simulink model "Perfect_blend_delayed_Quadcopter_Simulation"  (R2017a)
settings: Solver=ode45  StartTime=0.0  StopTime=35  FixedStep=0.05  MaxStep=0.06  RelTol=1e-3  EnableMultiTasking=on
model workspace (MAT data in the model file):
  Sig = Simulink.Signal
  Sig.DataType = 'auto'
  Sig.Dimensions = -1
  Sig.DimensionsMode = 'auto'
  Sig.Complexity = 'auto'
  Sig.SampleTime = -1
  Sig.SamplingMode = 'auto'
undefined symbols (not defined in the file or in its folder): altitude_error, blend_trigger, current_blend, error1, error2, error3, error4, IC, quadModel
libraries: simulink x4
(part 1 of 2)
Description:
  | This is a configurable quadcopter simulation.
  | This Simulink model demonstates position control.
  | 
  | Additional quadcopter modeling and simulation materials available at:
  | github.com/dch33/Quad-Sim
  | 
  | Copyright (C) 2014 D. Hartman, K. Landis, S. Moreno, J. Kim, M. Mehrer
  | 
  | License:
  |     This program is free software: you can redistribute it and/or modify
  |     it under the terms of the GNU LESSER GENERAL PUBLIC LICENSE as published by
  |     the Free Software Foundation, either version 3 of the License, or
  |     (at your option) any later version.
  | 
  |     This program is distributed in the hope that it will be useful,
  |     but WITHOUT ANY WARRANTY; without even the implied warranty of
  |     MERCHANTABILITY or FITNESS FOR A PARTICULAR PURPOSE.  See the
  |     GNU General Public License for more details.
  | 
  |     You should have received a copy of the GNU LESSER GENERAL PUBLIC LICENSE
  |     along with this program.  If not, see <http://www.gnu.org/licenses/>.
settings Model: ModifiedComment=davidhartman -- Fri Jun 06 22:59:54 2014 -- Version 1.5  Creator=David Hartman  LastModifiedBy=Yves
settings Model: ModifiedHistory=|
  | davidhartman -- Fri Jun 06 22:59:54 2014 -- Version 1.5
  | 
  | 
  | davidhartman -- Fri Jun 06 22:59:54 2014 -- Version 1.5
settings DataIOCC: ExternalInput=[Phi_sim_blend, Theta_sim_blend, Psi_sim_blend, error1, error2, error3, error4,]  FinalStateName=sim_result_final  InitialState=sim_state  SaveFormat=Array  SignalLogging=off  StateSaveName=sim_out_states  ReturnWorkspaceOutputsName=sim_all_outputs
settings OptimizationCC: DefaultParameterBehavior=Inlined  LifeSpan=inf
settings DebuggingCC: SolverPrmCheckMsg=warning  UniqueDataStoreMsg=warning  StateNameClashWarn=warning  StrictBusMsg=ErrorOnBusTreatedAsVector  SFUnexpectedBacktrackingDiag=warning  SFNoUnconditionalDefaultTransitionDiag=warning  SFExecutionAtInitializationDiag=none
settings HardwareCC: ProdBitPerPointer=32  ProdBitPerSizeT=32  ProdBitPerPtrDiffT=32  ProdLargestAtomicFloat=None  ProdIntDivRoundTo=Undefined  ProdEndianess=Unspecified  ProdWordSize=32  ProdHWDeviceType=32-bit Generic
settings ModelReferenceCC: PropagateSignalLabelsOutOfModel=off
settings GRTTargetCC: TargetLangStandard=C89/C90 (ANSI)  GeneratePreprocessorConditionals=Disable all
settings ConfigComp: CovMetricSettings=dw  CovHtmlReporting=on  CovSaveCumulativeToWorkspaceVar=on  CovSaveSingleToWorkspaceVar=on  CovExternalEMLEnable=off

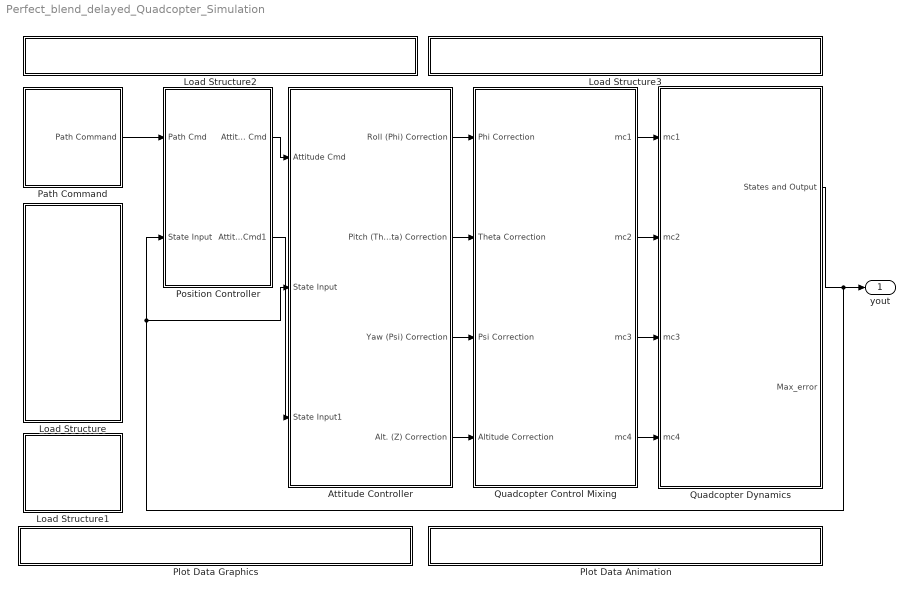
== system Perfect_blend_delayed_Quadcopter_Simulation ==
  Attitude Controller : Subsystem
  Load Structure : Subsystem
      settings: OpenFcn=|
      | uiopen('load')
      | if ((exist('IC')==1) && (exist('quadModel')==1) && (exist('path')==1))
      | set_param(bdroot, 'SimulationCommand', 'update')
      | end
      mask Display: fprintf('LOAD:\nTimeseries\nPath\nCommands,\nQuadcopter\nModel, Or\nInitial\nConditions');
  Load Structure1 : Subsystem
      settings: OpenFcn=|
      | if (exist('IC')==1 && exist('quadModel')==1 && exist('yout') && exist('tout'))
      | saveSimResults()
      | else
      | msgbox('No Data To Save!')
      | end
      mask Display: fprintf('SAVE:\nSimulation\nResults');
  Load Structure2 : Subsystem
      settings: OpenFcn=|
      | if exist('GUI_Modeling') == 2,
      | run('GUI_Modeling')
      | 
      | else
      | 
      | msgbox('The desired GUI must be first added to MATLABs path.')
      | 
      | end
      mask Display: fprintf('OPEN GUI: Build New \n Model');
  Load Structure3 : Subsystem
      settings: OpenFcn=|
      | if exist('GUI_IC') == 2,
      | run('GUI_IC')
      | 
      | else
      | 
      | msgbox('The desired GUI must be first added to MATLABs path.')
      | 
      | end
      mask Display: fprintf('OPEN GUI: Create Initial \n Conditions');
  Path Command : Subsystem  mask{Interpolate=on, OutputAfterFinalValue=Holding final value}
      mask prompts: Interpolate "Interpolate X, Y, Z, and Psi command data?"; OutputAfterFinalValue "Form output after final data value by:"
      mask help:
      | Selecting the Interpolate data checkbox causes position commands to be
      | linearly interpolated. For additional options related to the Timeseries
      | "path" commands, look under the block and click on the Timeseries From
      | Workspace blocks.
      mask TypeOptions Interpolate: X Timeseries From Wkspace/Interpolate | Y Timeseries From Wkspace/Interpolate | Z Timeseries From Wkspace/Interpolate | Psi Timeseries From Wkspace/Interpolate
      mask TypeOptions OutputAfterFinalValue: X Timeseries From Wkspace/OutputAfterFinalValue | Y Timeseries From Wkspace/OutputAfterFinalValue | Z Timeseries From Wkspace/OutputAfterFinalValue | Psi Timeseries From Wkspace/OutputAfterFinalValue
  Plot Data Animation : Subsystem
      settings: OpenFcn=|
      | if exist('QuadAnim4') == 2,
      |     if exist('yout')
      | 	run('QuadAnim4');
      |     else
      |     msgbox('Simulation must be run before data can be plotted.');
      |     end
      | else                                                                          msgbox('The desired GUI must be first added to MATLABs path.')
      | end
      mask Display: fprintf('OPEN GUI: Flight Animation')
  Plot Data Graphics : Subsystem
      settings: OpenFcn=|
      | if exist('yout')
      | yout = evalin('base', 'yout');
      | tout = evalin('base', 'tout');
      | quadPlots(yout, tout)
      | else
      | msgbox('Simulation must be run before data can be plotted.')
      | end
      mask Display: fprintf('OPEN PLOT: State Data')
  Position Controller : Subsystem
  Quadcopter Control Mixing : Subsystem
      mask Display:
      | modelLoaded = evalin('base','exist(''quadModel'',''var'')');
      | if (modelLoaded==1)
      |     if (evalin('base','quadModel.plusConfig'))
      |     fprintf([' \n' ' \n'  'Configuration "+"']);
      |     else if (~evalin('base','quadModel.plusConfig'))
      |         fprintf([' \n' ' \n' 'Configuration "X"']);
      |         end
      |     end
      | else
      |     fprintf([' \n' ' \n'  'Model Not Loaded']);
      | end
  Quadcopter Dynamics : Subsystem
  yout : Outport
  wires:
  Quadcopter Control Mixing/1(mc1) -> Quadcopter Dynamics/1(mc1)
  Quadcopter Control Mixing/2(mc2) -> Quadcopter Dynamics/2(mc2)
  Quadcopter Control Mixing/3(mc3) -> Quadcopter Dynamics/3(mc3)
  Quadcopter Control Mixing/4(mc4) -> Quadcopter Dynamics/4(mc4)
  Quadcopter Dynamics/1(States and Output) -> yout/1, Position Controller/2(State Input), Attitude Controller/2(State Input)
  Attitude Controller/1(Roll (Phi) Correction) -> Quadcopter Control Mixing/1(Phi Correction)
  Attitude Controller/2(Pitch (Theta) Correction) -> Quadcopter Control Mixing/2(Theta Correction)
  Attitude Controller/3(Yaw (Psi) Correction) -> Quadcopter Control Mixing/3(Psi Correction)
  Attitude Controller/4(Alt. (Z) Correction) -> Quadcopter Control Mixing/4(Altitude Correction)
  Path Command/1("Path Command ") -> Position Controller/1(Path Cmd)
  Position Controller/1(Attitude Cmd) -> Attitude Controller/1(Attitude Cmd)
  Position Controller/2(Attitude Cmd1) -> Attitude Controller/3(State Input1)

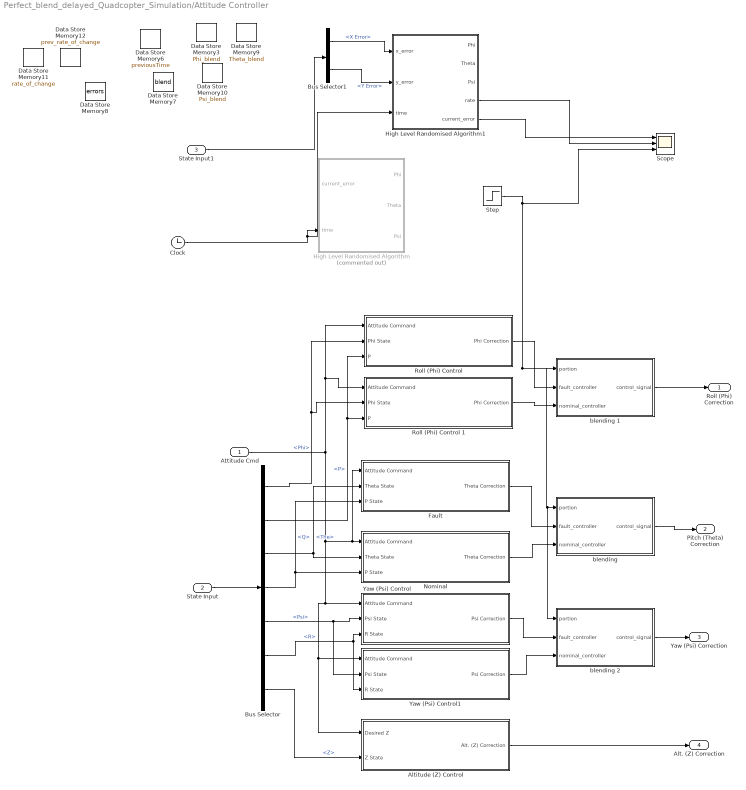
== system Perfect_blend_delayed_Quadcopter_Simulation/Attitude Controller ==
  Attitude Cmd : Inport
  State Input : Inport  Port=2
  State Input1 : Inport  Port=3
  Altitude (Z) Control : Subsystem  mask{Kpz=2, Kiz=1.1, Kdz=3.3, LimitOutput=on, USat=1, LSat=-1, GOffset=(sqrt((quadModel.mass*quadModel.g)/(4*quadModel.ct))-quadModel.b)/quadModel.cr}
      mask prompts: Kpz "Kp"; Kiz "Ki"; Kdz "Kd"; LimitOutput "Integral Saturation?"; USat "Upper saturation limit:"; LSat "Lower saturation limit:"; GOffset "Gravity Feedforward"
      mask help:
      | Adjust PID controller gains through this mask interface, or "look under mask" for more detailed adjustments.
      |
      | Note: Gravity Offset will not appear on block face as a value until simulation is run if it is the result of a formula involving the quadcopter model parameters.
      mask TypeOptions Kpz: Kpz/Gain
      mask TypeOptions Kiz: Kiz/Gain
      mask TypeOptions Kdz: Kdz/Gain
      mask TypeOptions LimitOutput:
      | Integrator
      | Limited/LimitOutput
      mask TypeOptions USat:
      | Integrator
      | Limited/UpperSaturationLimit
      mask TypeOptions LSat:
      | Integrator
      | Limited/LowerSaturationLimit
      mask TypeOptions GOffset: Gravity Offset (Level Flight)/Value
      mask Display:
      | fprintf(['Gravity Offset = ' num2str(GOffset) '\n' ...
      |     'Kp = ' num2str(Kpz) '\n' ...
      |     'Ki = ' num2str(Kiz) '\n' ...
      |     'Kd = ' num2str(Kdz) '\n' ...
      |     'Integral Saturation: ' LimitOutput]);
      | if strcmp(LimitOutput,'on')
      |     fprintf([' \n' ' \n' ' \n' ' \n' ' \n' '\n' ...
      |         'Limits: ' num2str(USat) ' to ' num2str(LSat)]);
      | end
  Bus Selector : BusSelector  OutputSignals=Phi,P,The,Q,Psi,R,Z
  Bus Selector1 : BusSelector  OutputSignals=X Error,Y Error
  Clock : Clock
  Data Store Memory10 : DataStoreMemory  DataStoreName=Psi_blend  ReadBeforeWriteMsg=warning  WriteAfterWriteMsg=warning  WriteAfterReadMsg=warning  ShowAdditionalParam=off  OutDataTypeStr=double
  Data Store Memory11 : DataStoreMemory  DataStoreName=rate_of_change  ReadBeforeWriteMsg=warning  WriteAfterWriteMsg=warning  WriteAfterReadMsg=warning  ShowAdditionalParam=off  OutDataTypeStr=double
  Data Store Memory12 : DataStoreMemory  DataStoreName=prev_rate_of_change  ReadBeforeWriteMsg=warning  WriteAfterWriteMsg=warning  WriteAfterReadMsg=warning  ShowAdditionalParam=off  OutDataTypeStr=double
  Data Store Memory3 : DataStoreMemory  DataStoreName=Phi_blend  ReadBeforeWriteMsg=warning  WriteAfterWriteMsg=warning  WriteAfterReadMsg=warning  ShowAdditionalParam=off  OutDataTypeStr=double
  Data Store Memory6 : DataStoreMemory  DataStoreName=previousTime  ReadBeforeWriteMsg=warning  WriteAfterWriteMsg=warning  WriteAfterReadMsg=warning  ShowAdditionalParam=off  OutDataTypeStr=double  Dimensions=[5 1]
  Data Store Memory7 : DataStoreMemory  DataStoreName=blend  ReadBeforeWriteMsg=warning  WriteAfterWriteMsg=warning  WriteAfterReadMsg=warning  ShowAdditionalParam=off  OutDataTypeStr=double
  Data Store Memory8 : DataStoreMemory  DataStoreName=errors  ReadBeforeWriteMsg=warning  WriteAfterWriteMsg=warning  WriteAfterReadMsg=warning  ShowAdditionalParam=off  OutDataTypeStr=double  Dimensions=[5 1]
  Data Store Memory9 : DataStoreMemory  DataStoreName=Theta_blend  ReadBeforeWriteMsg=warning  WriteAfterWriteMsg=warning  WriteAfterReadMsg=warning  ShowAdditionalParam=off  OutDataTypeStr=double
  Fault : Subsystem  mask{Kpt=10, Kit=5, Kdt=3, LimitOutput=on, USat=1, LSat=-1}
      mask prompts: Kpt "Kp"; Kit "Ki"; Kdt "Kd"; LimitOutput "Integral Saturation?"; USat "Upper saturation limit:"; LSat "Lower saturation limit:"
      mask help: Adjust PID controller gains through this mask interface, or "look under mask" for more detailed adjustments.
      mask TypeOptions Kpt: Kpt/Gain
      mask TypeOptions Kit: Kit/Gain
      mask TypeOptions Kdt: Kdt/Gain
      mask TypeOptions LimitOutput:
      | Integrator
      | Limited/LimitOutput
      mask TypeOptions USat:
      | Integrator
      | Limited/UpperSaturationLimit
      mask TypeOptions LSat:
      | Integrator
      | Limited/LowerSaturationLimit
      mask Display:
      | fprintf(['Kp = ' num2str(Kpt) '\n' ...
      |     'Ki = ' num2str(Kit) '\n' ...
      |     'Kd = ' num2str(Kdt) '\n' ...
      |     'Integral Saturation: ' LimitOutput]);
      | if strcmp(LimitOutput,'on')
      |     fprintf([' \n' ' \n' ' \n' ' \n' '\n' ...
      |         'Limits: ' num2str(USat) ' to ' num2str(LSat)]);
      | end
  High Level Randomised Algorithm : MATLAB Function  Commented=on  TreatAsAtomicUnit=on
  High Level Randomised Algorithm1 : MATLAB Function  TreatAsAtomicUnit=on
  Nominal : Subsystem  mask{Kpt=2, Kit=1.1, Kdt=1.2, LimitOutput=on, USat=1, LSat=-1}
      mask prompts: Kpt "Kp"; Kit "Ki"; Kdt "Kd"; LimitOutput "Integral Saturation?"; USat "Upper saturation limit:"; LSat "Lower saturation limit:"
      mask help: Adjust PID controller gains through this mask interface, or "look under mask" for more detailed adjustments.
      mask TypeOptions Kpt: Kpt/Gain
      mask TypeOptions Kit: Kit/Gain
      mask TypeOptions Kdt: Kdt/Gain
      mask TypeOptions LimitOutput:
      | Integrator
      | Limited/LimitOutput
      mask TypeOptions USat:
      | Integrator
      | Limited/UpperSaturationLimit
      mask TypeOptions LSat:
      | Integrator
      | Limited/LowerSaturationLimit
      mask Display:
      | fprintf(['Kp = ' num2str(Kpt) '\n' ...
      |     'Ki = ' num2str(Kit) '\n' ...
      |     'Kd = ' num2str(Kdt) '\n' ...
      |     'Integral Saturation: ' LimitOutput]);
      | if strcmp(LimitOutput,'on')
      |     fprintf([' \n' ' \n' ' \n' ' \n' '\n' ...
      |         'Limits: ' num2str(USat) ' to ' num2str(LSat)]);
      | end
  "Roll (Phi) Control " : Subsystem  mask{Kpp=10, Kip=5, Kdp=3, LimitOutput=on, USat=1, LSat=-1}
      mask prompts: Kpp "Kp"; Kip "Ki"; Kdp "Kd"; LimitOutput "Integral Saturation:"; USat "Upper saturation limit:"; LSat "Lower saturation limit:"
      mask help:
      | Adjust PID controller gains through this mask interface, or "look under mask"
      | for more detailed adjustments.
      mask TypeOptions Kpp: Kpp/Gain
      mask TypeOptions Kip: Kip/Gain
      mask TypeOptions Kdp: Kdp/Gain
      mask TypeOptions LimitOutput:
      | Integrator
      | Limited/LimitOutput
      mask TypeOptions USat:
      | Integrator
      | Limited/UpperSaturationLimit
      mask TypeOptions LSat:
      | Integrator
      | Limited/LowerSaturationLimit
      mask Display:
      | fprintf(['Kp = ' num2str(Kpp) '\n' ...
      |     'Ki = ' num2str(Kip) '\n' ...
      |     'Kd = ' num2str(Kdp) '\n'...
      |     'Integral Saturation: ' LimitOutput]);
      | if strcmp(LimitOutput,'on')
      |     fprintf([' \n' ' \n' ' \n' ' \n' '\n' ...
      |         'Limits: ' num2str(USat) ' to ' num2str(LSat)]);
      | end
  Roll (Phi) Control 1 : Subsystem  mask{Kpp=2.0, Kip=1.1, Kdp=1.2, LimitOutput=on, USat=1, LSat=-1}
      mask prompts: Kpp "Kp"; Kip "Ki"; Kdp "Kd"; LimitOutput "Integral Saturation:"; USat "Upper saturation limit:"; LSat "Lower saturation limit:"
      mask help:
      | Adjust PID controller gains through this mask interface, or "look under mask"
      | for more detailed adjustments.
      mask TypeOptions Kpp: Kpp/Gain
      mask TypeOptions Kip: Kip/Gain
      mask TypeOptions Kdp: Kdp/Gain
      mask TypeOptions LimitOutput:
      | Integrator
      | Limited/LimitOutput
      mask TypeOptions USat:
      | Integrator
      | Limited/UpperSaturationLimit
      mask TypeOptions LSat:
      | Integrator
      | Limited/LowerSaturationLimit
      mask Display:
      | fprintf(['Kp = ' num2str(Kpp) '\n' ...
      |     'Ki = ' num2str(Kip) '\n' ...
      |     'Kd = ' num2str(Kdp) '\n'...
      |     'Integral Saturation: ' LimitOutput]);
      | if strcmp(LimitOutput,'on')
      |     fprintf([' \n' ' \n' ' \n' ' \n' '\n' ...
      |         'Limits: ' num2str(USat) ' to ' num2str(LSat)]);
      | end
  Scope : Scope  NumInputPorts=3
  Step : Step  Time=blend_trigger  After=current_blend  SampleTime=0
  Yaw (Psi) Control : Subsystem  mask{Kps=12, Kis=2, Kds=5, LimitOutput=on, USat=1, LSat=-1}
      mask prompts: Kps "Kp"; Kis "Ki"; Kds "Kd"; LimitOutput "Integral Saturation?"; USat "Upper saturation limit:"; LSat "Lower saturation limit:"
      mask help: Adjust PID controller gains through this mask interface, or "look under mask" for more detailed adjustments.
      mask TypeOptions Kps: Kps/Gain
      mask TypeOptions Kis: Kit/Gain
      mask TypeOptions Kds: Kds/Gain
      mask TypeOptions LimitOutput:
      | Integrator
      | Limited/LimitOutput
      mask TypeOptions USat:
      | Integrator
      | Limited/UpperSaturationLimit
      mask TypeOptions LSat:
      | Integrator
      | Limited/LowerSaturationLimit
      mask Display:
      | fprintf(['Kp = ' num2str(Kps) '\n' ...
      |     'Ki = ' num2str(Kis) '\n' ...
      |     'Kd = ' num2str(Kds) '\n' ...
      |     'Integral Saturation: ' LimitOutput]);
      | if strcmp(LimitOutput,'on')
      |     fprintf([' \n' ' \n' ' \n' ' \n' '\n' ...
      |         'Limits: ' num2str(USat) ' to ' num2str(LSat)]);
      | end
  Yaw (Psi) Control1 : Subsystem  mask{Kps=4, Kis=0.5, Kds=3.5, LimitOutput=on, USat=1, LSat=-1}
      mask prompts: Kps "Kp"; Kis "Ki"; Kds "Kd"; LimitOutput "Integral Saturation?"; USat "Upper saturation limit:"; LSat "Lower saturation limit:"
      mask help: Adjust PID controller gains through this mask interface, or "look under mask" for more detailed adjustments.
      mask TypeOptions Kps: Kps/Gain
      mask TypeOptions Kis: Kit/Gain
      mask TypeOptions Kds: Kds/Gain
      mask TypeOptions LimitOutput:
      | Integrator
      | Limited/LimitOutput
      mask TypeOptions USat:
      | Integrator
      | Limited/UpperSaturationLimit
      mask TypeOptions LSat:
      | Integrator
      | Limited/LowerSaturationLimit
      mask Display:
      | fprintf(['Kp = ' num2str(Kps) '\n' ...
      |     'Ki = ' num2str(Kis) '\n' ...
      |     'Kd = ' num2str(Kds) '\n' ...
      |     'Integral Saturation: ' LimitOutput]);
      | if strcmp(LimitOutput,'on')
      |     fprintf([' \n' ' \n' ' \n' ' \n' '\n' ...
      |         'Limits: ' num2str(USat) ' to ' num2str(LSat)]);
      | end
  "blending " : MATLAB Function  TreatAsAtomicUnit=on
  blending 1 : MATLAB Function  TreatAsAtomicUnit=on
  blending 2 : MATLAB Function  TreatAsAtomicUnit=on
  Roll (Phi) Correction : Outport
  Pitch (Theta) Correction : Outport  Port=2
  Yaw (Psi) Correction : Outport  Port=3
  Alt. (Z) Correction : Outport  Port=4
  wires:
  Bus Selector/1 -> Roll (Phi) Control 1/2(Phi State), "Roll (Phi) Control "/2(Phi State)  "<Phi>"
  State Input/1 -> Bus Selector/1
  Bus Selector/5 -> Yaw (Psi) Control1/2(Psi State), Yaw (Psi) Control/2(Psi State)  "<Psi>"
  Altitude (Z) Control/1(Alt. (Z) Correction) -> Alt. (Z) Correction/1
  Bus Selector/7 -> Altitude (Z) Control/2(Z State)  "<Z>"
  Attitude Cmd/1 -> Yaw (Psi) Control1/1(Attitude Command), Altitude (Z) Control/1(Desired Z), Yaw (Psi) Control/1(Attitude Command), Fault/1(Attitude Command), Nominal/1(Attitude Command), Roll (Phi) Control 1/1("Attitude Command "), "Roll (Phi) Control "/1("Attitude Command ")
  Bus Selector/3 -> Nominal/2(Theta State), Fault/2(Theta State)  "<The>"
  Bus Selector/2 -> Roll (Phi) Control 1/3(P), "Roll (Phi) Control "/3(P)  "<P>"
  Bus Selector/4 -> Fault/3(P State), Nominal/3(P State)  "<Q>"
  Bus Selector/6 -> Yaw (Psi) Control1/3(R State), Yaw (Psi) Control/3(R State)  "<R>"
  Nominal/1(Theta Correction) -> "blending "/3(nominal_controller)
  Fault/1(Theta Correction) -> "blending "/2(fault_controller)
  "blending "/1(control_signal) -> Pitch (Theta) Correction/1
  Roll (Phi) Control 1/1(Phi Correction) -> blending 1/3(nominal_controller)
  "Roll (Phi) Control "/1(Phi Correction) -> blending 1/2(fault_controller)
  blending 1/1(control_signal) -> Roll (Phi) Correction/1
  Yaw (Psi) Control/1(Psi Correction) -> blending 2/2(fault_controller)
  Yaw (Psi) Control1/1(Psi Correction) -> blending 2/3(nominal_controller)
  blending 2/1(control_signal) -> Yaw (Psi) Correction/1
  Clock/1 -> High Level Randomised Algorithm1/3(time), High Level Randomised Algorithm/2(time)
  Step/1 -> Scope/3, blending 2/1(portion), "blending "/1(portion), blending 1/1(portion)
  Bus Selector1/2 -> High Level Randomised Algorithm1/2(y_error)  "<Y Error>"
  Bus Selector1/1 -> High Level Randomised Algorithm1/1(x_error)  "<X Error>"
  State Input1/1 -> Bus Selector1/1
  High Level Randomised Algorithm1/4(rate) -> Scope/2
  High Level Randomised Algorithm1/5(current_error) -> Scope/1

== system Perfect_blend_delayed_Quadcopter_Simulation/Load Structure ==

== system Perfect_blend_delayed_Quadcopter_Simulation/Load Structure1 ==

== system Perfect_blend_delayed_Quadcopter_Simulation/Load Structure2 ==

== system Perfect_blend_delayed_Quadcopter_Simulation/Load Structure3 ==

== system Perfect_blend_delayed_Quadcopter_Simulation/Path Command ==
  Bus Creator : BusCreator  Inputs=4
  Bus Selector : BusSelector  OutputSignals=X_cmd,Y_cmd  OutputAsBus=on
  Psi Timeseries From Wkspace : FromWorkspace  VariableName=path.psi  SampleTime=0  OutputAfterFinalValue=Holding final value
  X Timeseries From Wkspace : FromWorkspace  VariableName=path.x  SampleTime=0  OutputAfterFinalValue=Holding final value
  Y Timeseries From Wkspace : FromWorkspace  VariableName=path.y  SampleTime=0  OutputAfterFinalValue=Holding final value
  Z Timeseries From Wkspace : FromWorkspace  VariableName=path.z  SampleTime=0  OutputAfterFinalValue=Holding final value
  "Path Command " : Outport
  tag scope: C=global
  wires:
  X Timeseries From Wkspace/1 -> Bus Creator/1  "X_cmd"
  Y Timeseries From Wkspace/1 -> Bus Creator/2  "Y_cmd"
  Z Timeseries From Wkspace/1 -> Bus Creator/3  "Alt_Cmd"
  Psi Timeseries From Wkspace/1 -> Bus Creator/4  "Psi_cmd"
  Bus Creator/1 -> Bus Selector/1, "Path Command "/1  "Path_Cmd"
  Bus Selector/1 -> [C]  "XY_Cmd"

== system Perfect_blend_delayed_Quadcopter_Simulation/Plot Data Animation ==

== system Perfect_blend_delayed_Quadcopter_Simulation/Plot Data Graphics ==

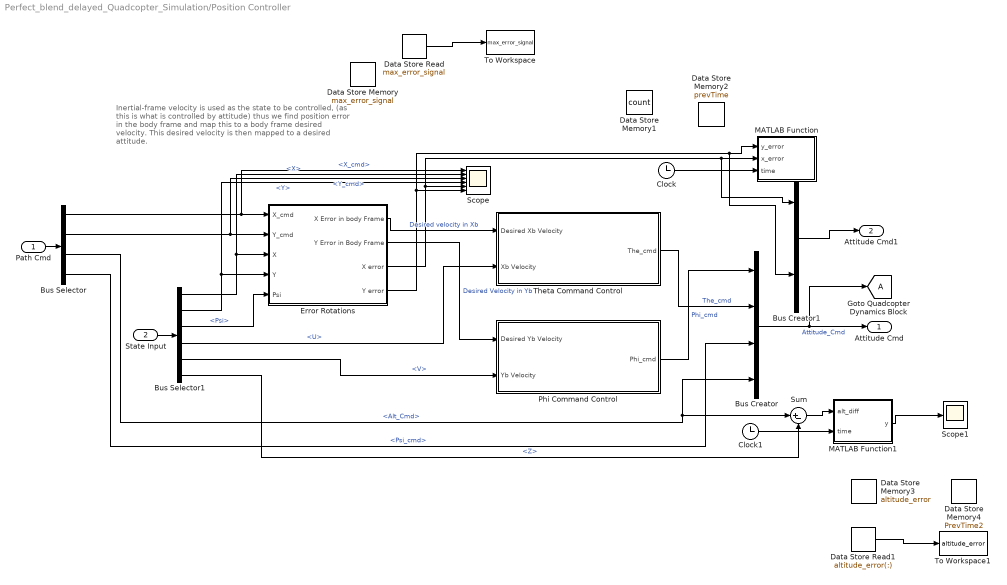
== system Perfect_blend_delayed_Quadcopter_Simulation/Position Controller ==
  note: Inertial-frame velocity is used as the state to be controlled,
      | (as this is what is controlled by attitude)
      | thus we find position error in the body frame
      | and map this to a body frame desired velocity. This desired
      | velocity is then mapped to a desired attitude.
  Path Cmd : Inport
  State Input : Inport  Port=2
  Bus Creator : BusCreator  Inputs=4
  Bus Creator1 : BusCreator  Inputs=2
  Bus Selector : BusSelector  OutputSignals=X_cmd,Y_cmd,Alt_Cmd,Psi_cmd
  Bus Selector1 : BusSelector  OutputSignals=X,Y,Psi,U,V,Z
  Clock : Clock
  Clock1 : Clock
  Data Store Memory : DataStoreMemory  DataStoreName=max_error_signal  ReadBeforeWriteMsg=warning  WriteAfterWriteMsg=warning  WriteAfterReadMsg=warning  ShowAdditionalParam=off  OutDataTypeStr=double
  Data Store Memory1 : DataStoreMemory  DataStoreName=count  ReadBeforeWriteMsg=warning  WriteAfterWriteMsg=warning  WriteAfterReadMsg=warning  ShowAdditionalParam=off  OutDataTypeStr=double
  Data Store Memory2 : DataStoreMemory  DataStoreName=prevTime  ReadBeforeWriteMsg=warning  WriteAfterWriteMsg=warning  WriteAfterReadMsg=warning  ShowAdditionalParam=off  OutDataTypeStr=double
  Data Store Memory3 : DataStoreMemory  DataStoreName=altitude_error  ReadBeforeWriteMsg=warning  WriteAfterWriteMsg=warning  WriteAfterReadMsg=warning  ShowAdditionalParam=off  OutDataTypeStr=double
  Data Store Memory4 : DataStoreMemory  DataStoreName=PrevTime2  ReadBeforeWriteMsg=warning  WriteAfterWriteMsg=warning  WriteAfterReadMsg=warning  ShowAdditionalParam=off  OutDataTypeStr=double
  Data Store Read : DataStoreRead  DataStoreName=max_error_signal  DataStoreElements=max_error_signal
  Data Store Read1 : DataStoreRead  DataStoreName=altitude_error  DataStoreElements=altitude_error(:)
  Error Rotations : Subsystem
  MATLAB Function : MATLAB Function  TreatAsAtomicUnit=on
  MATLAB Function1 : MATLAB Function  TreatAsAtomicUnit=on
  Phi Command Control : Subsystem  mask{Kp=0.32, Kd=0.1, ASat=12*pi/180}
      mask prompts: Kp "Proportional Gain"; Kd "Derivative Gain"; ASat "Attitude Limit (+/- radians):"
      mask TypeOptions Kp: Kpp/Gain
      mask TypeOptions Kd: Kdp/Gain
      mask TypeOptions ASat: Attitude Limits_Phi/UpperLimit
      mask Display:
      | fprintf(['Kp = ' num2str(Kp) '\n' ...
      |     'Kd = ' num2str(Kd) '\n' ...
      |     'Attitude Limit (+/-): ' num2str(ASat*180/pi) '°']);
  Scope : Scope  NumInputPorts=6
  Scope1 : Scope
  Sum : Sum  Inputs=|+-
  Theta Command Control : Subsystem  mask{Kp=0.32, Kd=0.10, ASat=12*pi/180}
      mask prompts: Kp "Proportional Gain:"; Kd "Derivative Gain"; ASat "Attitude Limit (+/- radians):"
      mask TypeOptions Kp: Kpt/Gain
      mask TypeOptions Kd: Kdt/Gain
      mask TypeOptions ASat: Attitude Limits_Theta/UpperLimit
      mask Display:
      | fprintf(['Kp = ' num2str(Kp) '\n' ...
      |     'Kd = ' num2str(Kd) '\n' ...
      |     'Attitude Limit (+/-): ' num2str(ASat*180/pi) '°']);
  To Workspace : ToWorkspace  VariableName=max_error_signal  SampleTime=-1
      settings: MaxDataPoints=1
  To Workspace1 : ToWorkspace  VariableName=altitude_error  SampleTime=-1
      settings: MaxDataPoints=1
  Attitude Cmd : Outport
  Attitude Cmd1 : Outport  Port=2
  tag scope: A=global
  wires:
  Bus Selector1/5 -> Phi Command Control/2(Yb Velocity)  "<V>"
  State Input/1 -> Bus Selector1/1
  Bus Selector/4 -> Bus Creator/3  "<Psi_cmd>"
  Path Cmd/1 -> Bus Selector/1
  Bus Selector/3 -> Sum/1, Bus Creator/4  "<Alt_Cmd>"
  Bus Creator/1 -> Attitude Cmd/1, [A]  "Attitude_Cmd"
  Bus Selector/1 -> Scope/1, Error Rotations/1(X_cmd)  "<X_cmd>"
  Bus Selector/2 -> Error Rotations/2(Y_cmd), Scope/3  "<Y_cmd>"
  Bus Selector1/1 -> Error Rotations/3(X), Scope/2  "<X>"
  Bus Selector1/2 -> Error Rotations/4(Y), Scope/4  "<Y>"
  Bus Selector1/3 -> Error Rotations/5(Psi)  "<Psi>"
  Error Rotations/1(X Error in body Frame) -> Theta Command Control/1(Desired Xb Velocity)  "Desired velocity in Xb"
  Bus Selector1/4 -> Theta Command Control/2(Xb Velocity)  "<U>"
  Theta Command Control/1(The_cmd) -> Bus Creator/2  "The_cmd"
  Error Rotations/2(Y Error in Body Frame) -> Phi Command Control/1(Desired Yb Velocity)  "Desired Velocity in Yb"
  Phi Command Control/1(Phi_cmd) -> Bus Creator/1  "Phi_cmd"
  Data Store Read/1 -> To Workspace/1
  Error Rotations/3(X error) -> Bus Creator1/1, MATLAB Function/2(x_error), Scope/5
  Error Rotations/4("Y error ") -> Bus Creator1/2, MATLAB Function/1(y_error), Scope/6
  Clock/1 -> MATLAB Function/3(time)
  MATLAB Function1/1(y) -> Scope1/1
  Data Store Read1/1 -> To Workspace1/1
  Sum/1 -> MATLAB Function1/1(alt_diff)
  Bus Selector1/6 -> Sum/2  "<Z>"
  Clock1/1 -> MATLAB Function1/2(time)
  Bus Creator1/1 -> Attitude Cmd1/1

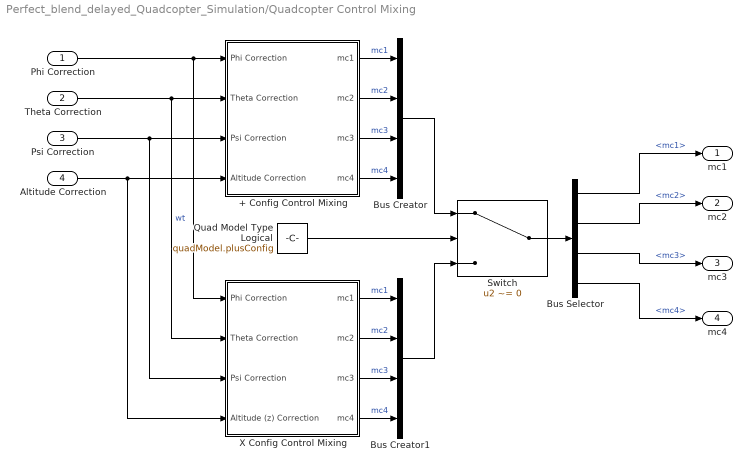
== system Perfect_blend_delayed_Quadcopter_Simulation/Quadcopter Control Mixing ==
  Phi Correction : Inport
  Theta Correction : Inport  Port=2
  Psi Correction : Inport  Port=3
  Altitude Correction : Inport  Port=4
  + Config Control Mixing : Subsystem
  Bus Creator : BusCreator  Inputs=4
  Bus Creator1 : BusCreator  Inputs=4
  Bus Selector : BusSelector  OutputSignals=mc1,mc2,mc3,mc4
  Quad Model Type Logical : Constant  Value=quadModel.plusConfig
  Switch : Switch  Criteria=u2 ~= 0
  X Config Control Mixing : Subsystem
  mc1 : Outport
  mc2 : Outport  Port=2
  mc3 : Outport  Port=3
  mc4 : Outport  Port=4
  wires:
  Phi Correction/1 -> X Config Control Mixing/1(Phi Correction), + Config Control Mixing/1(Phi Correction)
  Theta Correction/1 -> X Config Control Mixing/2(Theta Correction), + Config Control Mixing/2(Theta Correction)  "wt"
  Psi Correction/1 -> X Config Control Mixing/3(Psi Correction), + Config Control Mixing/3(Psi Correction)
  Altitude Correction/1 -> X Config Control Mixing/4(Altitude (z) Correction), + Config Control Mixing/4(Altitude Correction)
  + Config Control Mixing/1(mc1) -> Bus Creator/1  "mc1"
  + Config Control Mixing/2(mc2) -> Bus Creator/2  "mc2"
  + Config Control Mixing/3(mc3) -> Bus Creator/3  "mc3"
  + Config Control Mixing/4(mc4) -> Bus Creator/4  "mc4"
  Bus Creator/1 -> Switch/1
  X Config Control Mixing/1(mc1) -> Bus Creator1/1  "mc1"
  X Config Control Mixing/2(mc2) -> Bus Creator1/2  "mc2"
  X Config Control Mixing/3(mc3) -> Bus Creator1/3  "mc3"
  X Config Control Mixing/4(mc4) -> Bus Creator1/4  "mc4"
  Bus Creator1/1 -> Switch/3
  Bus Selector/1 -> mc1/1  "<mc1>"
  Bus Selector/2 -> mc2/1  "<mc2>"
  Bus Selector/3 -> mc3/1  "<mc3>"
  Bus Selector/4 -> mc4/1  "<mc4>"
  Quad Model Type Logical/1 -> Switch/2
  Switch/1 -> Bus Selector/1

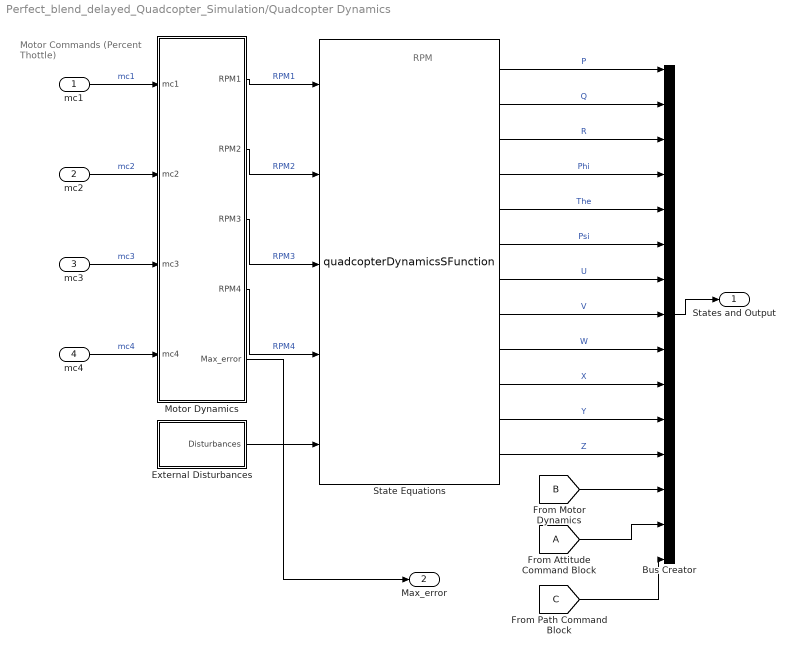
== system Perfect_blend_delayed_Quadcopter_Simulation/Quadcopter Dynamics ==
  note: RPM
  note: Motor Commands
      | (Percent Thottle)
  mc1 : Inport
  mc2 : Inport  Port=2
  mc3 : Inport  Port=3
  mc4 : Inport  Port=4
  Bus Creator : BusCreator  Inputs='P','Q','R','Phi','The','Psi','U','V','W','X','Y','Z','mc and RPM','Attitude_Cmd','XY_Cmd'
  External Disturbances : Subsystem
  Motor Dynamics : Subsystem
  State Equations : M-S-Function  FunctionName=quadcopterDynamicsSFunction  Parameters=quadModel, IC
      mask Display:
      | port_label('input', 1, 'RPM1')
      | port_label('input', 2, 'RPM2')
      | port_label('input', 3, 'RPM3')
      | port_label('input', 4, 'RPM4')
      | port_label('input', 5, 'Disturbances')
      | port_label('output', 1, 'P')
      | port_label('output', 2, 'Q')
      | port_label('output', 3, 'R')
      | port_label('output', 4, 'Phi')
      | port_label('output', 5, 'The')
      | port_label('output', 6, 'Psi')
      | port_label('output', 7, 'U')
      | port_label('output', 8, 'V')
      | port_label('output', 9, 'W')
      | port_label('output', 10, 'X')
      | port_label('output', 11, 'Y')
      | port_label('output', 12, 'Z')
  States and Output : Outport
  "Max_error " : Outport  Port=2
  wires:
  State Equations/1 -> Bus Creator/1  "P"
  State Equations/2 -> Bus Creator/2  "Q"
  State Equations/3 -> Bus Creator/3  "R"
  State Equations/4 -> Bus Creator/4  "Phi"
  State Equations/5 -> Bus Creator/5  "The"
  State Equations/6 -> Bus Creator/6  "Psi"
  State Equations/7 -> Bus Creator/7  "U"
  State Equations/8 -> Bus Creator/8  "V"
  State Equations/9 -> Bus Creator/9  "W"
  State Equations/10 -> Bus Creator/10  "X"
  State Equations/11 -> Bus Creator/11  "Y"
  State Equations/12 -> Bus Creator/12  "Z"
  Bus Creator/1 -> States and Output/1
  Motor Dynamics/1(RPM1) -> State Equations/1  "RPM1"
  Motor Dynamics/2(RPM2) -> State Equations/2  "RPM2"
  Motor Dynamics/3(RPM3) -> State Equations/3  "RPM3"
  Motor Dynamics/4(RPM4) -> State Equations/4  "RPM4"
  mc1/1 -> Motor Dynamics/1(mc1)  "mc1"
  mc4/1 -> Motor Dynamics/4(mc4)  "mc4"
  mc3/1 -> Motor Dynamics/3(mc3)  "mc3"
  mc2/1 -> Motor Dynamics/2(mc2)  "mc2"
  External Disturbances/1("Disturbances ") -> State Equations/5
  [A] -> Bus Creator/14
  [B] -> Bus Creator/13
  [C] -> Bus Creator/15
  Motor Dynamics/5("Max_error ") -> "Max_error "/1

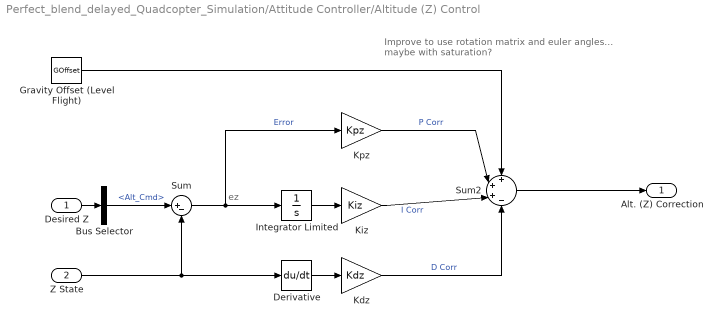
== system Perfect_blend_delayed_Quadcopter_Simulation/Attitude Controller/Altitude (Z) Control ==
  note: Improve to use rotation matrix and euler angles...
      | maybe with saturation?
  note: ez
  Desired Z : Inport
  Z State : Inport  Port=2
  Bus Selector : BusSelector  OutputSignals=Alt_Cmd
  Derivative : Derivative
  Gravity Offset (Level Flight) : Constant  Value=GOffset
  Integrator Limited : Integrator  LimitOutput=on  UpperSaturationLimit=USat  LowerSaturationLimit=LSat
  Kdz : Gain  Gain=Kdz
  Kiz : Gain  Gain=Kiz
  Kpz : Gain  Gain=Kpz
  Sum : Sum  Inputs=|+-
  Sum2 : Sum  Inputs=+++-
  Alt. (Z) Correction : Outport
  wires:
  Gravity Offset (Level Flight)/1 -> Sum2/1
  Desired Z/1 -> Bus Selector/1
  Z State/1 -> Derivative/1, Sum/2
  Sum2/1 -> Alt. (Z) Correction/1
  Kpz/1 -> Sum2/2  "P Corr"
  Sum/1 -> Integrator Limited/1, Kpz/1  "Error"
  Kiz/1 -> Sum2/3  "I Corr"
  Kdz/1 -> Sum2/4  "D Corr"
  Integrator Limited/1 -> Kiz/1
  Bus Selector/1 -> Sum/1  "<Alt_Cmd>"
  Derivative/1 -> Kdz/1

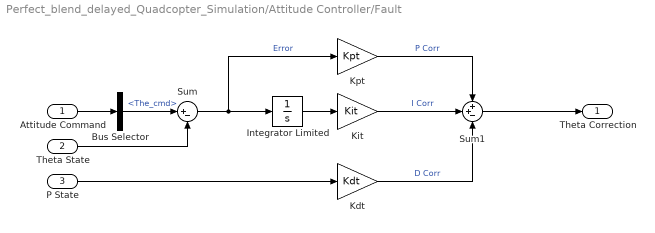
== system Perfect_blend_delayed_Quadcopter_Simulation/Attitude Controller/Fault ==
  Attitude Command : Inport
  Theta State : Inport  Port=2
  P State : Inport  Port=3
  Bus Selector : BusSelector  OutputSignals=The_cmd
  Integrator Limited : Integrator  LimitOutput=on  UpperSaturationLimit=USat  LowerSaturationLimit=LSat
  Kdt : Gain  Gain=Kdt
  Kit : Gain  Gain=Kit
  Kpt : Gain  Gain=Kpt
  Sum : Sum  Inputs=|+-
  Sum1 : Sum  Inputs=++-
  Theta Correction : Outport
  wires:
  Sum/1 -> Integrator Limited/1, Kpt/1  "Error"
  Attitude Command/1 -> Bus Selector/1
  Theta State/1 -> Sum/2
  Sum1/1 -> Theta Correction/1
  Kpt/1 -> Sum1/1  "P Corr"
  Kdt/1 -> Sum1/3  "D Corr"
  Kit/1 -> Sum1/2  "I Corr"
  Integrator Limited/1 -> Kit/1
  Bus Selector/1 -> Sum/1  "<The_cmd>"
  P State/1 -> Kdt/1

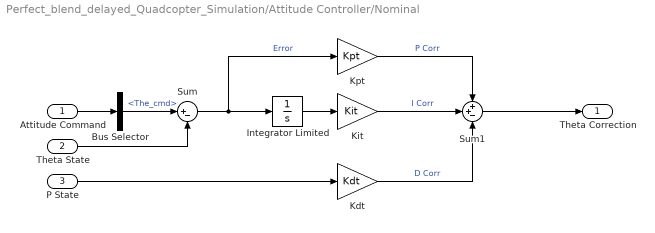
== system Perfect_blend_delayed_Quadcopter_Simulation/Attitude Controller/Nominal ==
  Attitude Command : Inport
  Theta State : Inport  Port=2
  P State : Inport  Port=3
  Bus Selector : BusSelector  OutputSignals=The_cmd
  Integrator Limited : Integrator  LimitOutput=on  UpperSaturationLimit=USat  LowerSaturationLimit=LSat
  Kdt : Gain  Gain=Kdt
  Kit : Gain  Gain=Kit
  Kpt : Gain  Gain=Kpt
  Sum : Sum  Inputs=|+-
  Sum1 : Sum  Inputs=++-
  Theta Correction : Outport
  wires:
  Sum/1 -> Integrator Limited/1, Kpt/1  "Error"
  Attitude Command/1 -> Bus Selector/1
  Theta State/1 -> Sum/2
  Sum1/1 -> Theta Correction/1
  Kpt/1 -> Sum1/1  "P Corr"
  Kdt/1 -> Sum1/3  "D Corr"
  Kit/1 -> Sum1/2  "I Corr"
  Integrator Limited/1 -> Kit/1
  Bus Selector/1 -> Sum/1  "<The_cmd>"
  P State/1 -> Kdt/1

== system Perfect_blend_delayed_Quadcopter_Simulation/Attitude Controller/Roll (Phi) Control  ==
  "Attitude Command " : Inport
  Phi State : Inport  Port=2
  P : Inport  Port=3
  Bus Selector : BusSelector  OutputSignals=Phi_cmd
  Integrator Limited : Integrator  LimitOutput=on  UpperSaturationLimit=USat  LowerSaturationLimit=LSat
  Kdp : Gain  Gain=Kdp
  Kip : Gain  Gain=Kip
  Kpp : Gain  Gain=Kpp
  Sum : Sum  Inputs=|+-
  Sum1 : Sum  Inputs=++-
  Phi Correction : Outport
  wires:
  Sum/1 -> Integrator Limited/1, Kpp/1  "Error"
  Phi State/1 -> Sum/2
  Sum1/1 -> Phi Correction/1
  Kpp/1 -> Sum1/1  "P Corr"
  Kdp/1 -> Sum1/3  "D Corr"
  Kip/1 -> Sum1/2  "I Corr"
  Integrator Limited/1 -> Kip/1
  "Attitude Command "/1 -> Bus Selector/1
  Bus Selector/1 -> Sum/1  "<Phi_cmd>"
  P/1 -> Kdp/1

== system Perfect_blend_delayed_Quadcopter_Simulation/Attitude Controller/Roll (Phi) Control 1 ==
  "Attitude Command " : Inport
  Phi State : Inport  Port=2
  P : Inport  Port=3
  Bus Selector : BusSelector  OutputSignals=Phi_cmd
  Integrator Limited : Integrator  LimitOutput=on  UpperSaturationLimit=USat  LowerSaturationLimit=LSat
  Kdp : Gain  Gain=Kdp
  Kip : Gain  Gain=Kip
  Kpp : Gain  Gain=Kpp
  Sum : Sum  Inputs=|+-
  Sum1 : Sum  Inputs=++-
  Phi Correction : Outport
  wires:
  P/1 -> Kdp/1
  Bus Selector/1 -> Sum/1  "<Phi_cmd>"
  "Attitude Command "/1 -> Bus Selector/1
  Integrator Limited/1 -> Kip/1
  Kip/1 -> Sum1/2  "I Corr"
  Kdp/1 -> Sum1/3  "D Corr"
  Kpp/1 -> Sum1/1  "P Corr"
  Sum1/1 -> Phi Correction/1
  Phi State/1 -> Sum/2
  Sum/1 -> Kpp/1, Integrator Limited/1  "Error"

== system Perfect_blend_delayed_Quadcopter_Simulation/Attitude Controller/Yaw (Psi) Control ==
  Attitude Command : Inport
  Psi State : Inport  Port=2
  R State : Inport  Port=3
  Bus Selector : BusSelector  OutputSignals=Psi_cmd
  Integrator Limited : Integrator  LimitOutput=on  UpperSaturationLimit=USat  LowerSaturationLimit=LSat
  Kds : Gain  Gain=Kds
  Kit : Gain  Gain=Kis
  Kps : Gain  Gain=Kps
  Sum : Sum  Inputs=|+-
  Sum1 : Sum  Inputs=++-
  Psi Correction : Outport
  wires:
  Sum/1 -> Integrator Limited/1, Kps/1  "Error"
  Attitude Command/1 -> Bus Selector/1
  Sum1/1 -> Psi Correction/1
  Psi State/1 -> Sum/2
  Kps/1 -> Sum1/1  "P Corr"
  Kds/1 -> Sum1/3  "D Corr"
  Kit/1 -> Sum1/2  "I Corr"
  Integrator Limited/1 -> Kit/1
  Bus Selector/1 -> Sum/1  "<Psi_cmd>"
  R State/1 -> Kds/1

== system Perfect_blend_delayed_Quadcopter_Simulation/Attitude Controller/Yaw (Psi) Control1 ==
  Attitude Command : Inport
  Psi State : Inport  Port=2
  R State : Inport  Port=3
  Bus Selector : BusSelector  OutputSignals=Psi_cmd
  Integrator Limited : Integrator  LimitOutput=on  UpperSaturationLimit=USat  LowerSaturationLimit=LSat
  Kds : Gain  Gain=Kds
  Kit : Gain  Gain=Kis
  Kps : Gain  Gain=Kps
  Sum : Sum  Inputs=|+-
  Sum1 : Sum  Inputs=++-
  Psi Correction : Outport
  wires:
  Sum/1 -> Integrator Limited/1, Kps/1  "Error"
  Attitude Command/1 -> Bus Selector/1
  Sum1/1 -> Psi Correction/1
  Psi State/1 -> Sum/2
  Kps/1 -> Sum1/1  "P Corr"
  Kds/1 -> Sum1/3  "D Corr"
  Kit/1 -> Sum1/2  "I Corr"
  Integrator Limited/1 -> Kit/1
  Bus Selector/1 -> Sum/1  "<Psi_cmd>"
  R State/1 -> Kds/1

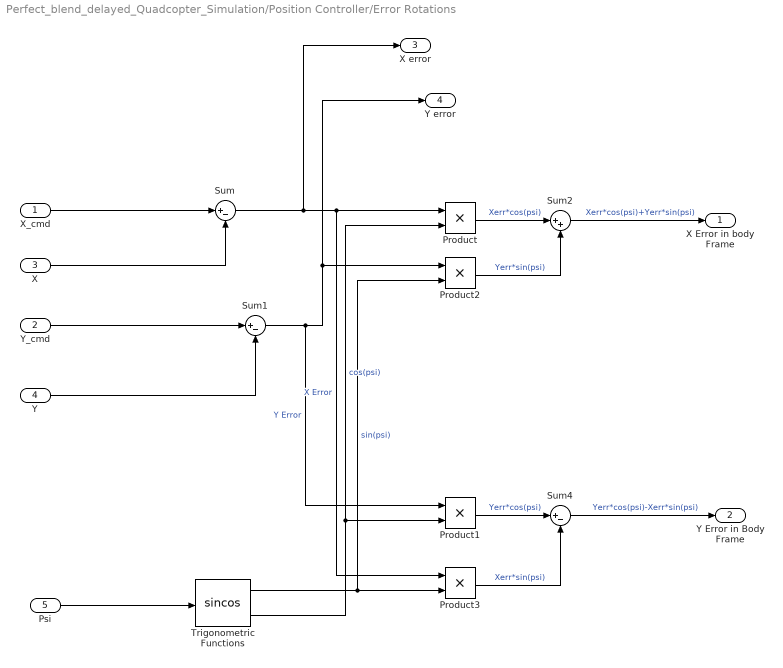
== system Perfect_blend_delayed_Quadcopter_Simulation/Position Controller/Error Rotations ==
  X_cmd : Inport
  Y_cmd : Inport  Port=2
  X : Inport  Port=3
  Y : Inport  Port=4
  Psi : Inport  Port=5
  Product{,1..3} (4 alike) : Product
  Sum : Sum  Inputs=|+-
  Sum1 : Sum  Inputs=|+-
  Sum2 : Sum  Inputs=|++
  Sum4 : Sum  Inputs=|+-
  Trigonometric Functions : Trigonometry  Operator=sincos
  X Error in body Frame : Outport
  Y Error in Body Frame : Outport  Port=2
  X error : Outport  Port=3
  "Y error " : Outport  Port=4
  wires:
  Sum4/1 -> Y Error in Body Frame/1  "Yerr*cos(psi)-Xerr*sin(psi)"
  Product3/1 -> Sum4/2  "Xerr*sin(psi)"
  Sum1/1 -> "Y error "/1, Product2/1, Product1/1  "Y Error"
  Trigonometric Functions/1 -> Product2/2, Product3/2  "sin(psi)"
  Sum2/1 -> X Error in body Frame/1  "Xerr*cos(psi)+Yerr*sin(psi)"
  Y_cmd/1 -> Sum1/1
  X_cmd/1 -> Sum/1
  X/1 -> Sum/2
  Y/1 -> Sum1/2
  Sum/1 -> X error/1, Product3/1, Product/1  "X Error"
  Trigonometric Functions/2 -> Product/2, Product1/2  "cos(psi)"
  Product/1 -> Sum2/1  "Xerr*cos(psi)"
  Product2/1 -> Sum2/2  "Yerr*sin(psi)"
  Product1/1 -> Sum4/1  "Yerr*cos(psi)"
  Psi/1 -> Trigonometric Functions/1

== system Perfect_blend_delayed_Quadcopter_Simulation/Position Controller/Phi Command Control ==
  note: -1 Gain is required because a "negative"
      | angle of Phi induces a positive velocity
      | in the body frame y direction!
  Desired Yb Velocity : Inport
  Yb Velocity : Inport  Port=2
  Attitude Limits_Phi : Saturate  UpperLimit=ASat  LowerLimit=-ASat
  Gain : Gain  Gain=-1
  Kdp : Gain  Gain=Kd
  Kpp : Gain  Gain=Kp
  Sum3 : Sum  Inputs=|+-
  Sum6 : Sum  Inputs=|+-
  V Derivative : Derivative
  Phi_cmd : Outport
  wires:
  V Derivative/1 -> Kdp/1
  Attitude Limits_Phi/1 -> Phi_cmd/1  "Phi_cmd"
  Sum6/1 -> Gain/1
  Kpp/1 -> Sum6/1
  Sum3/1 -> Kpp/1  "Velocity Error"
  Yb Velocity/1 -> V Derivative/1, Sum3/2
  Desired Yb Velocity/1 -> Sum3/1
  Gain/1 -> Attitude Limits_Phi/1
  Kdp/1 -> Sum6/2

== system Perfect_blend_delayed_Quadcopter_Simulation/Position Controller/Theta Command Control ==
  Desired Xb Velocity : Inport
  Xb Velocity : Inport  Port=2
  Attitude Limits_Theta : Saturate  UpperLimit=ASat  LowerLimit=-ASat
  Kdt : Gain  Gain=Kd
  Kpt : Gain  Gain=Kp
  Sum3 : Sum  Inputs=|+-
  Sum6 : Sum  Inputs=|+-
  U Derivative : Derivative
  The_cmd : Outport
  wires:
  Kdt/1 -> Sum6/2
  U Derivative/1 -> Kdt/1
  Attitude Limits_Theta/1 -> The_cmd/1  "The_cmd"
  Sum6/1 -> Attitude Limits_Theta/1
  Kpt/1 -> Sum6/1
  Sum3/1 -> Kpt/1  "Velocity Error"
  Xb Velocity/1 -> U Derivative/1, Sum3/2
  Desired Xb Velocity/1 -> Sum3/1

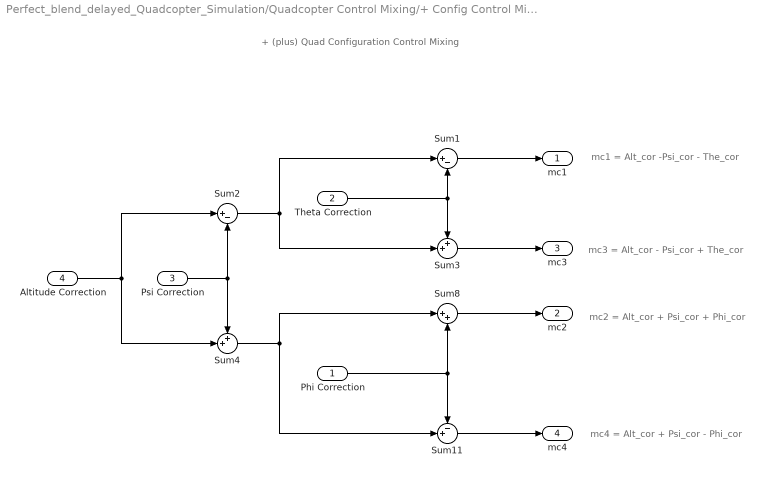
== system Perfect_blend_delayed_Quadcopter_Simulation/Quadcopter Control Mixing/+ Config Control Mixing ==
  note: mc2 = Alt_cor + Psi_cor + Phi_cor
  note: + (plus) Quad Configuration Control Mixing
  note: mc4 = Alt_cor + Psi_cor - Phi_cor
  note: mc3 = Alt_cor - Psi_cor + The_cor
  note: mc1 = Alt_cor -Psi_cor - The_cor
  Phi Correction : Inport
  Theta Correction : Inport  Port=2
  Psi Correction : Inport  Port=3
  Altitude Correction : Inport  Port=4
  Sum1 : Sum  Inputs=|+-
  Sum11 : Sum  Inputs=-+|
  Sum2 : Sum  Inputs=|+-
  Sum3 : Sum  Inputs=++|
  Sum4 : Sum  Inputs=++|
  Sum8 : Sum  Inputs=|++
  mc1 : Outport
  mc2 : Outport  Port=2
  mc3 : Outport  Port=3
  mc4 : Outport  Port=4
  wires:
  Altitude Correction/1 -> Sum2/1, Sum4/2
  Sum2/1 -> Sum3/2, Sum1/1
  Psi Correction/1 -> Sum4/1, Sum2/2
  Sum4/1 -> Sum11/2, Sum8/1
  Phi Correction/1 -> Sum8/2, Sum11/1
  Sum1/1 -> mc1/1
  Sum3/1 -> mc3/1
  Sum8/1 -> mc2/1
  Sum11/1 -> mc4/1
  Theta Correction/1 -> Sum1/2, Sum3/1

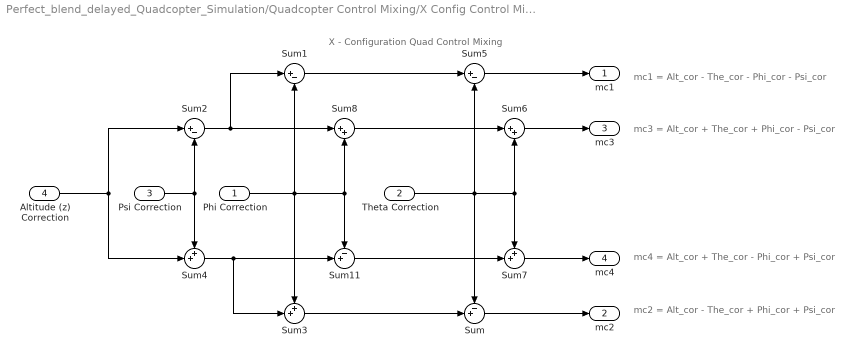
== system Perfect_blend_delayed_Quadcopter_Simulation/Quadcopter Control Mixing/X Config Control Mixing ==
  note: mc1 = Alt_cor - The_cor - Phi_cor - Psi_cor
  note: X - Configuration Quad Control Mixing
  note: mc3 = Alt_cor + The_cor + Phi_cor - Psi_cor
  note: mc2 = Alt_cor - The_cor + Phi_cor + Psi_cor
  note: mc4 = Alt_cor + The_cor - Phi_cor + Psi_cor
  Phi Correction : Inport
  Theta Correction : Inport  Port=2
  Psi Correction : Inport  Port=3
  Altitude (z) Correction : Inport  Port=4
  Sum : Sum  Inputs=-+|
  Sum1 : Sum  Inputs=|+-
  Sum11 : Sum  Inputs=-+|
  Sum2 : Sum  Inputs=|+-
  Sum3 : Sum  Inputs=++|
  Sum4 : Sum  Inputs=++|
  Sum5 : Sum  Inputs=|+-
  Sum6 : Sum  Inputs=|++
  Sum7 : Sum  Inputs=++|
  Sum8 : Sum  Inputs=|++
  mc1 : Outport
  mc2 : Outport  Port=2
  mc3 : Outport  Port=3
  mc4 : Outport  Port=4
  wires:
  Sum2/1 -> Sum8/1, Sum1/1
  Psi Correction/1 -> Sum4/1, Sum2/2
  Phi Correction/1 -> Sum3/1, Sum1/2, Sum8/2, Sum11/1
  Sum4/1 -> Sum3/2, Sum11/2
  Sum3/1 -> Sum/2
  Theta Correction/1 -> Sum7/1, Sum6/2, Sum5/2, Sum/1
  Sum1/1 -> Sum5/1
  Sum8/1 -> Sum6/1
  Sum11/1 -> Sum7/2
  Sum5/1 -> mc1/1
  Sum6/1 -> mc3/1
  Sum7/1 -> mc4/1
  Altitude (z) Correction/1 -> Sum2/1, Sum4/2
  Sum/1 -> mc2/1

== system Perfect_blend_delayed_Quadcopter_Simulation/Quadcopter Dynamics/External Disturbances ==
  note: Note: Torques are in units of N*m, Forces in N
      | Torques are applied to the BODY coordinate system.
      | Forces are applied from the WORLD coordinate system!
      | This can be changed by adjusting the equations within the S-function.
  Bus Creator : BusCreator  Inputs=6
  Bus to Vector : BusToVector
  Constant{2..6} (5 alike) : Constant  Value=0
  Step : Step  After=0  SampleTime=0
  "Disturbances " : Outport
  wires:
  Bus to Vector/1 -> "Disturbances "/1
  Bus Creator/1 -> Bus to Vector/1
  Constant6/1 -> Bus Creator/1  "Tau_bx-axis"
  Step/1 -> Bus Creator/2  "Tau_by-axis"
  Constant2/1 -> Bus Creator/3  "Tau_bz-axis"
  Constant3/1 -> Bus Creator/4  "Force_x-axis"
  Constant4/1 -> Bus Creator/5  "Force_y-axis"
  Constant5/1 -> Bus Creator/6  "Force_z-axis"

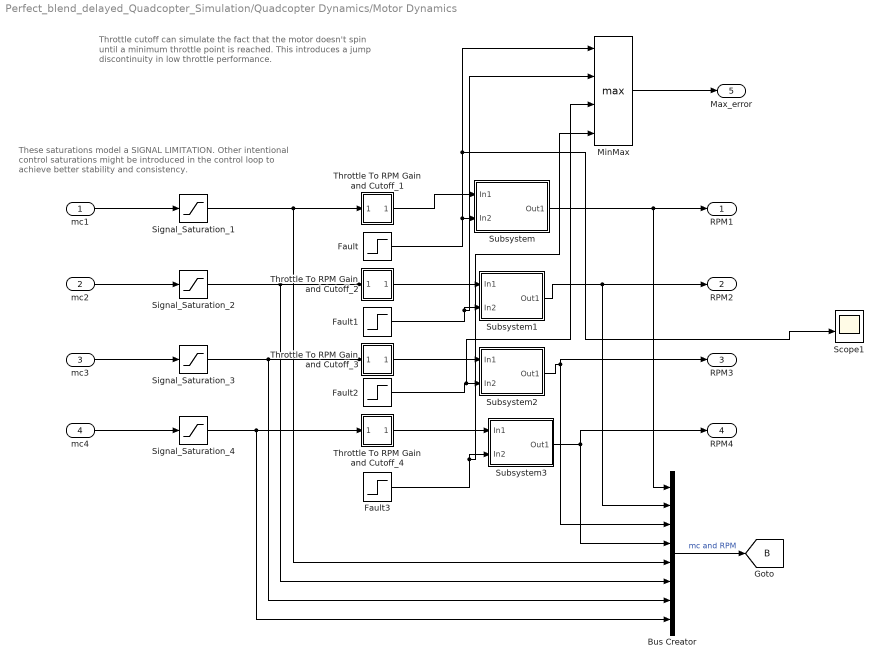
== system Perfect_blend_delayed_Quadcopter_Simulation/Quadcopter Dynamics/Motor Dynamics ==
  note: Throttle cutoff can simulate the fact that the motor doesn't
      | spin until a minimum throttle point is reached. This introduces
      | a jump discontinuity in low throttle performance.
  note: These saturations model a SIGNAL LIMITATION.
      | Other intentional control saturations might be introduced in the
      | control loop to achieve better stability and consistency.
  mc1 : Inport
  mc2 : Inport  Port=2
  mc3 : Inport  Port=3
  mc4 : Inport  Port=4
  Bus Creator : BusCreator  Inputs=8
  Fault : Step  Time=15  After=error1  SampleTime=0
  Fault1 : Step  Time=15  After=error2  SampleTime=0
  Fault2 : Step  Time=15  After=error3  SampleTime=0
  Fault3 : Step  Time=15  After=error4  SampleTime=0
  MinMax : MinMax  Function=max  Inputs=4
  Scope1 : Scope  NumInputPorts=4
  Signal_Saturation_{1..4} (4 alike) : Saturate  UpperLimit=100  LowerLimit=0
  Subsystem : Subsystem
  Subsystem1 : Subsystem
  Subsystem2 : Subsystem
  Subsystem3 : Subsystem
  Throttle To RPM Gain and Cutoff_1 : Subsystem
  Throttle To RPM Gain and Cutoff_2 : Subsystem
  Throttle To RPM Gain and Cutoff_3 : Subsystem
  Throttle To RPM Gain and Cutoff_4 : Subsystem
  RPM1 : Outport
  RPM2 : Outport  Port=2
  RPM3 : Outport  Port=3
  RPM4 : Outport  Port=4
  "Max_error " : Outport  Port=5
  tag scope: B=global
  wires:
  mc1/1 -> Signal_Saturation_1/1
  mc4/1 -> Signal_Saturation_4/1
  mc2/1 -> Signal_Saturation_2/1
  mc3/1 -> Signal_Saturation_3/1
  Signal_Saturation_1/1 -> Bus Creator/5, Throttle To RPM Gain and Cutoff_1/1(In5)
  Signal_Saturation_2/1 -> Bus Creator/6, Throttle To RPM Gain and Cutoff_2/1(In5)
  Signal_Saturation_3/1 -> Bus Creator/7, Throttle To RPM Gain and Cutoff_3/1(In5)
  Signal_Saturation_4/1 -> Bus Creator/8, Throttle To RPM Gain and Cutoff_4/1(In5)
  Throttle To RPM Gain and Cutoff_4/1(Out5) -> Subsystem3/1(In1)
  Subsystem3/1(Out1) -> RPM4/1, Bus Creator/4
  Bus Creator/1 -> [B]  "mc and RPM"
  Subsystem/1(Out1) -> Bus Creator/1, RPM1/1
  Throttle To RPM Gain and Cutoff_1/1(Out5) -> Subsystem/1(In1)
  Fault/1 -> Scope1/3, MinMax/1, Subsystem/2(In2)
  Subsystem2/1(Out1) -> Bus Creator/3, RPM3/1
  Subsystem1/1(Out1) -> Bus Creator/2, RPM2/1
  Throttle To RPM Gain and Cutoff_2/1(Out5) -> Subsystem1/1(In1)
  Throttle To RPM Gain and Cutoff_3/1(Out5) -> Subsystem2/1(In1)
  Fault2/1 -> MinMax/3, Subsystem2/2(In2)
  Fault3/1 -> MinMax/4, Subsystem3/2(In2)
  Fault1/1 -> MinMax/2, Subsystem1/2(In2)
  MinMax/1 -> "Max_error "/1

== system Perfect_blend_delayed_Quadcopter_Simulation/Quadcopter Dynamics/Motor Dynamics/Subsystem ==
  In1 : Inport
  In2 : Inport  Port=2
  MATLAB Function : MATLAB Function  TreatAsAtomicUnit=on
  Motor_Dynamics_1 : StateSpace  A=-1/quadModel.T  C=1/quadModel.T  D=0  X0=IC.w1*quadModel.T
  Scope : Scope  NumInputPorts=4
  Out1 : Outport
  wires:
  In1/1 -> Motor_Dynamics_1/1
  MATLAB Function/1(rotor_speed) -> Scope/3, Out1/1
  In2/1 -> MATLAB Function/1(fault)
  Motor_Dynamics_1/1 -> Scope/2, MATLAB Function/2(nominal_model_input)

== system Perfect_blend_delayed_Quadcopter_Simulation/Quadcopter Dynamics/Motor Dynamics/Subsystem1 ==
  In1 : Inport
  In2 : Inport  Port=2
  MATLAB Function : MATLAB Function  TreatAsAtomicUnit=on
  "Motor_Dynamics_2 " : StateSpace  A=-1/quadModel.T  C=1/quadModel.T  D=0  X0=IC.w1*quadModel.T
  Out1 : Outport
  wires:
  In1/1 -> "Motor_Dynamics_2 "/1
  MATLAB Function/1(rotor_speed) -> Out1/1
  In2/1 -> MATLAB Function/1(fault)
  "Motor_Dynamics_2 "/1 -> MATLAB Function/2(nominal_modal_input)

== system Perfect_blend_delayed_Quadcopter_Simulation/Quadcopter Dynamics/Motor Dynamics/Subsystem2 ==
  In1 : Inport
  In2 : Inport  Port=2
  MATLAB Function : MATLAB Function  TreatAsAtomicUnit=on
  "Motor_Dynamics_3 " : StateSpace  A=-1/quadModel.T  C=1/quadModel.T  D=0  X0=IC.w1*quadModel.T
  Out1 : Outport
  wires:
  In1/1 -> "Motor_Dynamics_3 "/1
  MATLAB Function/1(rotor_speed) -> Out1/1
  In2/1 -> MATLAB Function/1(fault)
  "Motor_Dynamics_3 "/1 -> MATLAB Function/2(nominal_modal_input)

== system Perfect_blend_delayed_Quadcopter_Simulation/Quadcopter Dynamics/Motor Dynamics/Subsystem3 ==
  In1 : Inport
  In2 : Inport  Port=2
  MATLAB Function : MATLAB Function  TreatAsAtomicUnit=on
  "Motor_Dynamics_4 " : StateSpace  A=-1/quadModel.T  C=1/quadModel.T  D=0  X0=IC.w1*quadModel.T
  Out1 : Outport
  wires:
  In1/1 -> "Motor_Dynamics_4 "/1
  MATLAB Function/1(rotor_speed) -> Out1/1
  In2/1 -> MATLAB Function/1(fault)
  "Motor_Dynamics_4 "/1 -> MATLAB Function/2(nominal_modal_input)

== system Perfect_blend_delayed_Quadcopter_Simulation/Quadcopter Dynamics/Motor Dynamics/Throttle To RPM Gain and Cutoff_1 ==
  note: minThr should be a quad.mat value
  note: This gain should be a quad.mat value
  note: This constant should be a quad.mat value
  note: Output equals linearly scaled RPM
      | for given throttle input if throttle input >=Throttle Cuttoff (minThr)
      | else output is zero.
  In5 : Inport
  Constant : Constant  Value=quadModel.b
  Gain : Gain  Gain=quadModel.cr
  Minimum Throttle Cutoff : simulink/Logic and Bit Operations/Compare To Constant  relop=>=  const=quadModel.minThr  OutDataTypeStr=uint8
  Product : Product
  Sum1 : Sum  Inputs=++|
  Out5 : Outport
  wires:
  Minimum Throttle Cutoff/1 -> Product/2
  Product/1 -> Out5/1
  In5/1 -> Gain/1, Minimum Throttle Cutoff/1
  Gain/1 -> Sum1/2
  Sum1/1 -> Product/1
  Constant/1 -> Sum1/1

== system Perfect_blend_delayed_Quadcopter_Simulation/Quadcopter Dynamics/Motor Dynamics/Throttle To RPM Gain and Cutoff_2 ==
  note: minThr should be a quad.mat value
  note: This gain should be a quad.mat value
  note: This constant should be a quad.mat value
  note: Output equals linearly scaled RPM
      | for given throttle input if throttle input >=Throttle Cuttoff (minThr)
      | else output is zero.
  In5 : Inport
  Constant : Constant  Value=quadModel.b
  Gain : Gain  Gain=quadModel.cr
  Minimum Throttle Cutoff : simulink/Logic and Bit Operations/Compare To Constant  relop=>=  const=quadModel.minThr  OutDataTypeStr=uint8
  Product : Product
  Sum1 : Sum  Inputs=++|
  Out5 : Outport
  wires:
  Minimum Throttle Cutoff/1 -> Product/2
  Product/1 -> Out5/1
  In5/1 -> Gain/1, Minimum Throttle Cutoff/1
  Gain/1 -> Sum1/2
  Sum1/1 -> Product/1
  Constant/1 -> Sum1/1

== system Perfect_blend_delayed_Quadcopter_Simulation/Quadcopter Dynamics/Motor Dynamics/Throttle To RPM Gain and Cutoff_3 ==
  note: minThr should be a quad.mat value
  note: This gain should be a quad.mat value
  note: This constant should be a quad.mat value
  note: Output equals linearly scaled RPM
      | for given throttle input if throttle input >=Throttle Cuttoff (minThr)
      | else output is zero.
  In5 : Inport
  Constant : Constant  Value=quadModel.b
  Gain : Gain  Gain=quadModel.cr
  Minimum Throttle Cutoff : simulink/Logic and Bit Operations/Compare To Constant  relop=>=  const=quadModel.minThr  OutDataTypeStr=uint8
  Product : Product
  Sum1 : Sum  Inputs=++|
  Out5 : Outport
  wires:
  Minimum Throttle Cutoff/1 -> Product/2
  Product/1 -> Out5/1
  In5/1 -> Gain/1, Minimum Throttle Cutoff/1
  Gain/1 -> Sum1/2
  Sum1/1 -> Product/1
  Constant/1 -> Sum1/1
